simulink model "PMSM_model_2018b"  (R2017b)
settings: Solver=ode15s  StartTime=0.0  StopTime=1  FixedStep=0.0001  RelTol=1e-3
InitFcn:
  | r=1.2
  | Ld=5.7*10^-3
  | Lq=12.5*10^-3
  | PM=123*10^-3
  | P=4
  | b=0
  | J=0.0001
libraries: fl_lib x5, nesl_utility x4, pe_lib x3
settings Model: Creator=Aliraqe  LastModifiedBy=Aliraqe

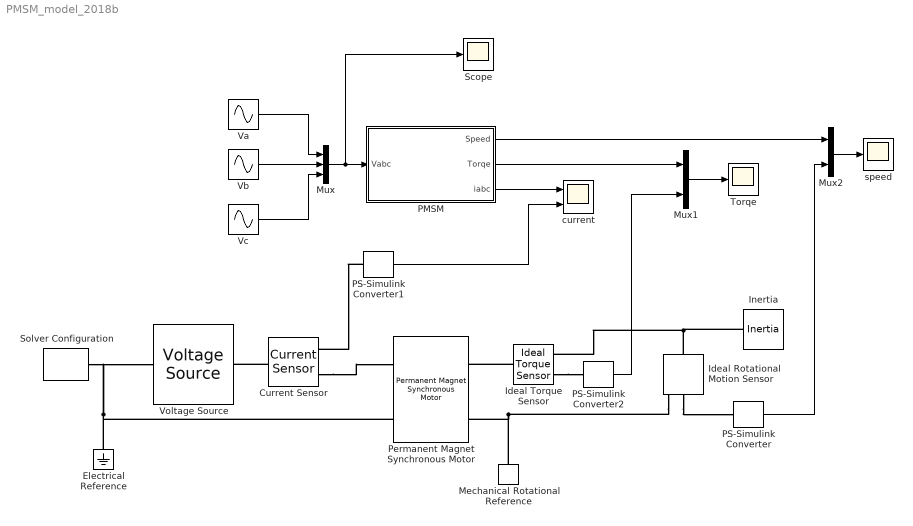
== system PMSM_model_2018b ==
  Current Sensor : pe_lib/Sensors/Current Sensor
      settings: SourceProductName=Simscape Power Systems  SourceProductBaseCode=PS
  Electrical Reference : fl_lib/Electrical/Electrical Elements/Electrical Reference
  Ideal Rotational Motion Sensor : fl_lib/Mechanical/Mechanical Sensors/Ideal Rotational Motion Sensor  offset=0 deg
      settings: SourceProductName=Foundation Library
  Ideal Torque Sensor : fl_lib/Mechanical/Mechanical Sensors/Ideal Torque Sensor
      settings: SourceProductName=Foundation Library
  Inertia : fl_lib/Mechanical/Rotational Elements/Inertia  inertia="0.0001  kg*m^2"  w_specify=off  w_priority=High  w=0 rad/s  w_nominal_specify=off  w_nominal_unit=rad/s  w_nominal_value=1  t_specify=off  t_priority=None  t=0 N*m  t_nominal_specify=off  t_nominal_unit=N*m  t_nominal_value=1
  Mechanical Rotational Reference : fl_lib/Mechanical/Rotational Elements/Mechanical Rotational Reference
  Mux : Mux  Inputs=3
  Mux1 : Mux  Inputs=2
  Mux2 : Mux  Inputs=2
  PMSM : Subsystem
  PS-Simulink Converter : nesl_utility/PS-Simulink Converter  PhysicalDomain=network_engine_domain  SubClassName=ps_output  LeftPortType=input  RightPortType=output  PseudoPeriodic=off  Frequencies=[]  Unit=rad/s  AffineConversion=off
  PS-Simulink Converter1 : nesl_utility/PS-Simulink Converter  PhysicalDomain=network_engine_domain  SubClassName=ps_output  LeftPortType=input  RightPortType=output  PseudoPeriodic=off  Frequencies=[]  Unit=A  AffineConversion=off
  PS-Simulink Converter2 : nesl_utility/PS-Simulink Converter  PhysicalDomain=network_engine_domain  SubClassName=ps_output  LeftPortType=input  RightPortType=output  PseudoPeriodic=off  Frequencies=[]  Unit=N*m  AffineConversion=off
  Permanent Magnet Synchronous Motor : pe_lib/Machines/Permanent Magnet Rotor/Permanent Magnet Synchronous Motor  nPolePairs=P/2  pmflux_param=1  pm_flux_linkage=PM Wb  torque_constant=0.18 N*m/A  back_emf_constant=0.18 V/(rad/s)  stator_param=1  Ld=Ld H  Lq=Lq H  L0=0 H  Ls=0.0002 H  Lm=-0.00002 H  Ms=0.00002 H  Rs=r Ohm  initial_currents=[0, 0, 0] A  axes_param=2  angular_position0=0 deg  rotor_offset=-pi / 2 rad  shift_3ph=[nan, nan, nan] rad  sqrt2OverSqrt3=nan  oneOverSqrt2=nan  twoPiOver3=nan  Lmin=1e-9 H
      settings: SourceProductName=Simscape Power Systems  SourceProductBaseCode=PS
  Scope : Scope
  Solver Configuration : nesl_utility/Solver Configuration  PhysicalDomain=network_engine_domain  SubClassName=solver  LeftPortType=input  RightPortType=generic  Accelerate=off  Tones=[]  Harmonics=[]  SimulateNoise=off  Profile=off  UseLocalSampling=off  EnableSwitchedLinearOptims=on  FrequencyDomain=off  UseCCode=off  RelTol=0.001  AbsTol=1e-06  MinStep=1e-09  ToWorkspace=off  RevertToSquareIcSolve=off  NumHomotopyIterations=100  PhasorMode=off  PhasorModeNumHarmonics=1  DoDC=off  ResidualTolerance=1e-09  UseLocalSolver=off  LocalSolverChoice=NE_BACKWARD_EULER_ADVANCER  LocalSolverSampleTime=0.001  DoFixedCost=off  MaxNonlinIter=3  MaxModeIter=2  LinearAlgebra=Sparse  DelaysMemoryBudget=1024  AutomaticFiltering=on  FilteringTimeConstant=0.001
  "Torqe " : Scope
  Va : Sin  Amplitude=220*sqrt(2)  Frequency=2*pi*60  SampleTime=0
  Vb : Sin  Amplitude=220*sqrt(2)  Frequency=2*pi*60  Phase=-2*pi/3  SampleTime=0
  Vc : Sin  Amplitude=220*sqrt(2)  Frequency=2*pi*60  Phase=2*pi/3  SampleTime=0
  Voltage Source : pe_lib/Sources/Voltage Source  vline_rms=380 V  shift=0 deg  freq=60 Hz  impedance_option=0  SShortCircuit=1e6 V*A  XR=15  R=0.01 Ohm  L=3.97e-4 H  G_parasitic=0 1/Ohm  harmonic_option=0  harmonic_orders=[5, 7, 11, 13]  harmonic_ratios=[.1, .1, .1, .1]  I_specify=off  I_priority=None  I=[ 0 0 0 ] A  I_nominal_specify=off  I_nominal_unit=A  I_nominal_value=1
      settings: SourceProductName=Simscape Power Systems  SourceProductBaseCode=PS
  current : Scope  NumInputPorts=2
  speed : Scope
  wires:
  Va/1 -> Mux/1
  Vb/1 -> Mux/2
  Vc/1 -> Mux/3
  Mux/1 -> Scope/1, PMSM/1(Vabc)
  PMSM/1("Speed ") -> Mux2/1
  Mux2/1 -> speed/1
  PS-Simulink Converter2/1 -> Mux1/2
  PS-Simulink Converter/1 -> Mux2/2
  PMSM/2(Torqe) -> Mux1/1
  Mux1/1 -> "Torqe "/1
  PS-Simulink Converter1/1 -> current/2
  PMSM/3(iabc) -> current/1
  connections:
  Electrical Reference/LConn1 -- Permanent Magnet Synchronous Motor/LConn2 -- Voltage Source/LConn1 -- Solver Configuration/RConn1
  Inertia/LConn1 -- Ideal Rotational Motion Sensor/LConn1 -- Ideal Torque Sensor/RConn1
  Ideal Torque Sensor/LConn1 -- Permanent Magnet Synchronous Motor/RConn1
  Ideal Torque Sensor/RConn2 -- PS-Simulink Converter2/LConn1
  Ideal Rotational Motion Sensor/RConn2 -- PS-Simulink Converter/LConn1
  Mechanical Rotational Reference/LConn1 -- Ideal Rotational Motion Sensor/RConn1 -- Permanent Magnet Synchronous Motor/RConn2
  Current Sensor/LConn1 -- Voltage Source/RConn1
  Current Sensor/RConn2 -- Permanent Magnet Synchronous Motor/LConn1
  PS-Simulink Converter1/LConn1 -- Current Sensor/RConn1

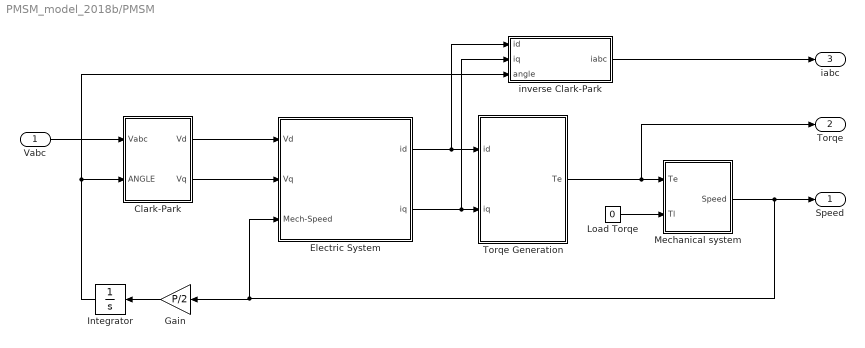
== system PMSM_model_2018b/PMSM ==
  Vabc : Inport
  Clark-Park : Subsystem
  "Electric System " : Subsystem
  Gain : Gain  Gain=P/2
  Integrator : Integrator
  Load Torqe : Constant  Value=0
  Mechanical system : Subsystem
  Torqe Generation : Subsystem
  inverse Clark-Park : Subsystem
  "Speed " : Outport
  Torqe : Outport  Port=2
  iabc : Outport  Port=3
  wires:
  Load Torqe/1 -> Mechanical system/2(Tl)
  Clark-Park/1(Vd) -> "Electric System "/1(Vd)
  Torqe Generation/1(Te) -> Torqe/1, Mechanical system/1(Te)
  Clark-Park/2(Vq) -> "Electric System "/2("Vq ")
  Mechanical system/1(Speed) -> "Speed "/1, "Electric System "/3("Mech-Speed "), Gain/1
  "Electric System "/1("id ") -> Torqe Generation/1(id), inverse Clark-Park/1(id)
  Vabc/1 -> Clark-Park/1(Vabc)
  "Electric System "/2(iq) -> inverse Clark-Park/2(iq), Torqe Generation/2("iq ")
  Gain/1 -> Integrator/1
  Integrator/1 -> inverse Clark-Park/3(angle), Clark-Park/2("ANGLE ")
  inverse Clark-Park/1(iabc) -> iabc/1

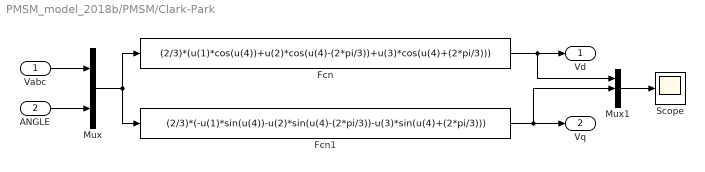
== system PMSM_model_2018b/PMSM/Clark-Park ==
  Vabc : Inport
  "ANGLE " : Inport  Port=2
  Fcn : Fcn  Expr=(2/3)*(u(1)*cos(u(4))+u(2)*cos(u(4)-(2*pi/3))+u(3)*cos(u(4)+(2*pi/3)))
  Fcn1 : Fcn  Expr=(2/3)*(-u(1)*sin(u(4))-u(2)*sin(u(4)-(2*pi/3))-u(3)*sin(u(4)+(2*pi/3)))
  Mux : Mux  Inputs=2
  Mux1 : Mux  Inputs=3
  Scope : Scope
  Vd : Outport
  Vq : Outport  Port=2
  wires:
  Fcn/1 -> Mux1/1, Vd/1
  Vabc/1 -> Mux/1
  Mux/1 -> Fcn1/1, Fcn/1
  Fcn1/1 -> Mux1/2, Vq/1
  Mux1/1 -> Scope/1
  "ANGLE "/1 -> Mux/2

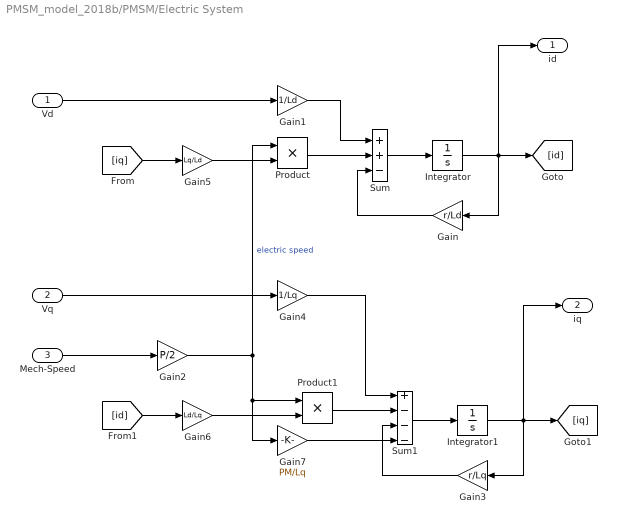
== system PMSM_model_2018b/PMSM/Electric System  ==
  Vd : Inport
  "Vq " : Inport  Port=2
  "Mech-Speed " : Inport  Port=3
  Gain : Gain  Gain=r/Ld
  Gain1 : Gain  Gain=1/Ld
  Gain2 : Gain  Gain=P/2
  Gain3 : Gain  Gain=r/Lq
  Gain4 : Gain  Gain=1/Lq
  Gain5 : Gain  Gain=Lq/Ld
  Gain6 : Gain  Gain=Ld/Lq
  Gain7 : Gain  Gain=PM/Lq
  Integrator : Integrator
  Integrator1 : Integrator
  Product : Product
  Product1 : Product
  Sum : Sum  Inputs=++-
  Sum1 : Sum  Inputs=+---
  "id " : Outport
  iq : Outport  Port=2
  wires:
  Integrator/1 -> "id "/1, [id], Gain/1
  Gain1/1 -> Sum/1
  Sum/1 -> Integrator/1
  Vd/1 -> Gain1/1
  Gain/1 -> Sum/3
  Product/1 -> Sum/2
  Gain3/1 -> Sum1/3
  Gain4/1 -> Sum1/1
  Product1/1 -> Sum1/2
  "Vq "/1 -> Gain4/1
  Sum1/1 -> Integrator1/1
  Integrator1/1 -> iq/1, [iq], Gain3/1
  "Mech-Speed "/1 -> Gain2/1
  Gain2/1 -> Gain7/1, Product1/1, Product/1  "electric speed"
  [iq] -> Gain5/1
  Gain5/1 -> Product/2
  [id] -> Gain6/1
  Gain6/1 -> Product1/2
  Gain7/1 -> Sum1/4

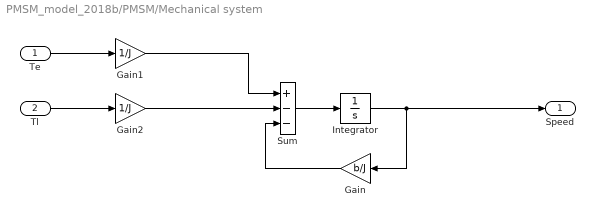
== system PMSM_model_2018b/PMSM/Mechanical system ==
  Te : Inport
  Tl : Inport  Port=2
  Gain : Gain  Gain=b/J
  Gain1 : Gain  Gain=1/J
  Gain2 : Gain  Gain=1/J
  Integrator : Integrator
  Sum : Sum  Inputs=+--
  Speed : Outport
  wires:
  Integrator/1 -> Speed/1, Gain/1
  Gain1/1 -> Sum/1
  Gain2/1 -> Sum/2
  Sum/1 -> Integrator/1
  Gain/1 -> Sum/3
  Te/1 -> Gain1/1
  Tl/1 -> Gain2/1

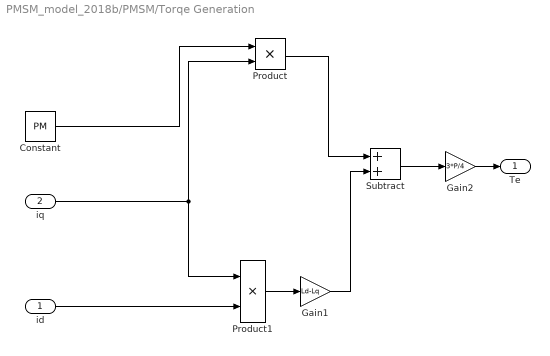
== system PMSM_model_2018b/PMSM/Torqe Generation ==
  id : Inport
  "iq " : Inport  Port=2
  Constant : Constant  Value=PM
  Gain1 : Gain  Gain=Ld-Lq
  Gain2 : Gain  Gain=3*P/4
  Product : Product
  Product1 : Product
  Subtract : Sum
  Te : Outport
  wires:
  id/1 -> Product1/2
  Constant/1 -> Product/1
  "iq "/1 -> Product1/1, Product/2
  Product/1 -> Subtract/1
  Subtract/1 -> Gain2/1
  Gain2/1 -> Te/1
  Product1/1 -> Gain1/1
  Gain1/1 -> Subtract/2

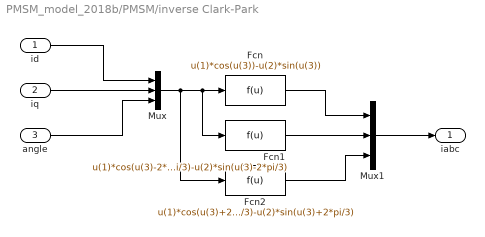
== system PMSM_model_2018b/PMSM/inverse Clark-Park ==
  id : Inport
  iq : Inport  Port=2
  angle : Inport  Port=3
  Fcn : Fcn  Expr=u(1)*cos(u(3))-u(2)*sin(u(3))
  Fcn1 : Fcn  Expr=u(1)*cos(u(3)-2*pi/3)-u(2)*sin(u(3)-2*pi/3)
  Fcn2 : Fcn  Expr=u(1)*cos(u(3)+2*pi/3)-u(2)*sin(u(3)+2*pi/3)
  Mux : Mux  Inputs=3
  Mux1 : Mux  Inputs=3
  iabc : Outport
  wires:
  id/1 -> Mux/1
  iq/1 -> Mux/2
  angle/1 -> Mux/3
  Mux/1 -> Fcn2/1, Fcn1/1, Fcn/1
  Fcn/1 -> Mux1/1
  Fcn1/1 -> Mux1/2
  Fcn2/1 -> Mux1/3
  Mux1/1 -> iabc/1
